simulink model "dT_test"  (R2019b)
settings: Solver=ode3  StartTime=0.0  StopTime=30  MaxStep=0.5  MinStep=0.1  RelTol=1e-3
values from neighbouring files (symbols this model uses):
  cube = sim('cubesat_propagation' ,[0 1])    [SCARSSetup.m]    (also in plot_position.m = sim('cubesat_propagation' ,[TStart TFinal]); pwsat2_setup.m; scars_setup.m)
  dT = dT2    [SCARSSetup.m]    (also in plot_position.m = 0.1; pwsat2_setup.m = 5; scars_setup.m = 0.1; startup.m = 1)
  initEuler = [0 0 0]    [SCARSSetup.m]    (also in pwsat2_setup.m; scars_setup.m)
undefined symbols (not defined in the file or in its folder): Earth, WGS84
libraries: aerolib6dof2 x1, sharedtransform x1, aerolibgravity2 x1, aerolibutil x1
settings Model: Creator=asmialek  LastModifiedBy=asmialek
settings SolverCC: MaxConsecutiveZCs=2
settings DebuggingCC: TimeAdjustmentMsg=warning  SolverPrmCheckMsg=warning  InheritedTsInSrcMsg=error  SingleTaskRateTransMsg=error  SigSpecEnsureSampleTimeMsg=error  FixptConstUnderflowMsg=warning  FixptConstOverflowMsg=warning  FixptConstPrecisionLossMsg=warning  UnnecessaryDatatypeConvMsg=warning  VectorMatrixConversionMsg=warning  SignalLabelMismatchMsg=warning  SFcnCompatibilityMsg=warning  ModelReferenceIOMsg=warning  ModelReferenceVersionMismatchMessage=warning  ModelReferenceIOMismatchMessage=warning  StateNameClashWarn=warning  StrictBusMsg=WarnOnBusTreatedAsVector  NonBusSignalsTreatedAsBus=warning

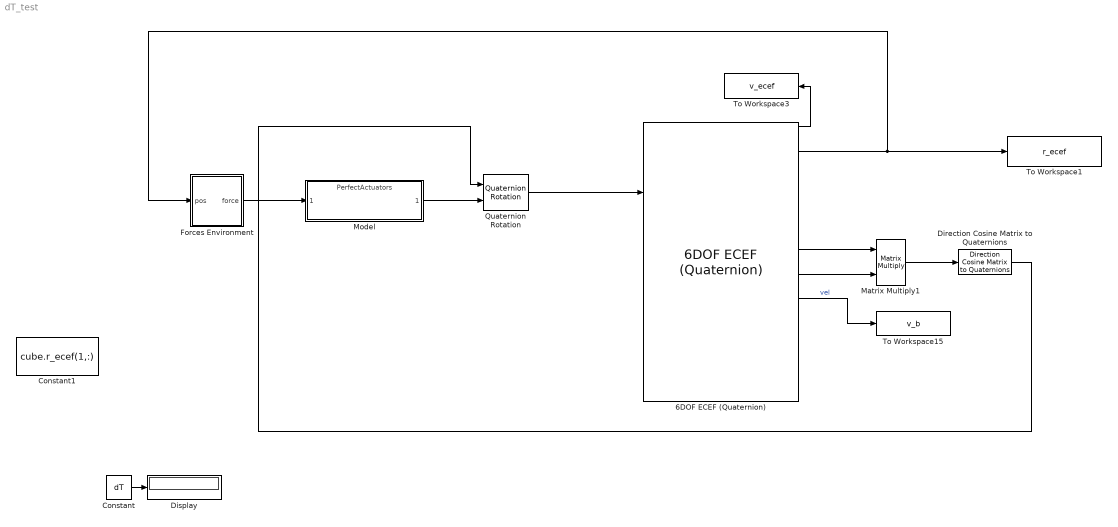
== system dT_test ==
  6DOF ECEF (Quaternion) : aerolib6dof2/6DOF ECEF (Quaternion)  units=Metric (MKS)  mtype=Fixed  xg_0=r_lla  Vm_0=v_b  eul_0=deg2rad(initEuler)  pm_0=[0 0 0]  mass_0=1.0  mass_e=0.5  mass_f=2.0  inertia=eye(3)  inertia_e=eye(3)  inertia_f=2*eye(3)  vre_flag=on  abi_flag=off  ptype=Earth (WGS84)  R=6378137  F=1/298.257223563  w_E=7292115e-11  angle_in=Internal  LG0=0  quat_statename=''  pm_statename=''  Vm_statename=''  posECEF_statename=''  posECI_statename=''  LG_statename=''  mass_statename=''
      settings: SourceProductName=Aerospace Blockset  SourceProductBaseCode=AE
  Constant : Constant  Value=dT
  Constant1 : Constant  Value=cube.r_ecef(1,:)
  Direction Cosine Matrix to Quaternions : sharedtransform/Direction Cosine Matrix  to Quaternions  aMode=0  action=None  tolerance=eps(2)
      settings: SourceProductName=Aerospace Blockset  SourceProductBaseCode=AE
  Display : Display
  Forces Environment : Subsystem
  Matrix Multiply1 : Product  Multiplication=Matrix(*)
  Model : ModelReference  ModelNameDialog=PerfectActuators.slx  SimulationMode=Normal  ModelReferenceVersion=1.7
  Quaternion Rotation : aerolibutil/Quaternion Rotation
  To Workspace1 : ToWorkspace  VariableName=r_ecef  SampleTime=-1
  To Workspace15 : ToWorkspace  VariableName=v_b  SampleTime=-1
      settings: Save2DSignal=2-D array (concatenate along first dimension)
  To Workspace3 : ToWorkspace  VariableName=v_ecef  SampleTime=-1
      settings: Save2DSignal=2-D array (concatenate along first dimension)
  wires:
  Constant/1 -> Display/1
  6DOF ECEF (Quaternion)/6 -> Matrix Multiply1/1
  Direction Cosine Matrix to Quaternions/1 -> Quaternion Rotation/1
  6DOF ECEF (Quaternion)/8 -> To Workspace15/1  "vel"
  Quaternion Rotation/1 -> 6DOF ECEF (Quaternion)/1
  Forces Environment/1(force) -> Model/1
  6DOF ECEF (Quaternion)/7 -> Matrix Multiply1/2
  6DOF ECEF (Quaternion)/1 -> To Workspace3/1
  Matrix Multiply1/1 -> Direction Cosine Matrix to Quaternions/1
  6DOF ECEF (Quaternion)/2 -> Forces Environment/1(pos), To Workspace1/1
  Model/1 -> Quaternion Rotation/2

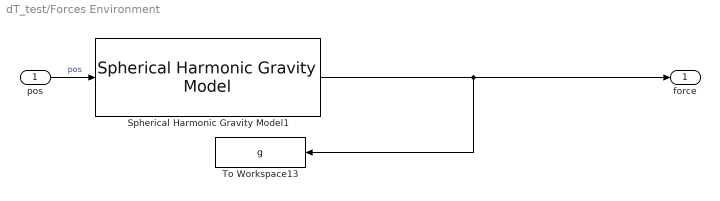
== system dT_test/Forces Environment ==
  pos : Inport
  Spherical Harmonic Gravity Model1 : aerolibgravity2/Spherical Harmonic Gravity Model  units=Metric (MKS)  degree=120  action=Error  ptype=EGM2008  datafile='aerogmm2b.mat'
      settings: SourceProductName=Aerospace Blockset  SourceProductBaseCode=AE
  To Workspace13 : ToWorkspace  VariableName=g  SampleTime=-1
  force : Outport
  wires:
  Spherical Harmonic Gravity Model1/1 -> force/1, To Workspace13/1
  pos/1 -> Spherical Harmonic Gravity Model1/1  "pos"
